simulink model "IPC"  (R2019b)
settings: Solver=FixedStepAuto  StartTime=0.0  StopTime=10  FixedStep=0.1  RelTol=1e-3
settings Model: Creator=JDALUZ1  LastModifiedBy=EMORAI12
settings SolverCC: PositivePriorityOrder=on  AutoInsertRateTranBlk=on  InsertRTBMode=Always
settings DebuggingCC: ArithmeticOperatorsInVariantConditions=warning
settings SFSimCC: CustomCodeUndefinedFunction=UseInterfaceOnly
settings CodeAppCC: StateflowObjectComments=on

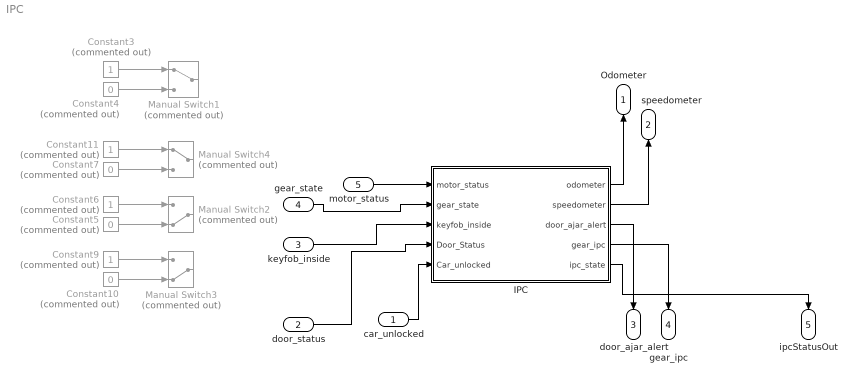
== system IPC ==
  car_unlocked : Inport
  door_status : Inport  Port=2
  keyfob_inside : Inport  Port=3
  gear_state : Inport  Port=4
  motor_status : Inport  Port=5
  Constant{4..5,7,10} (4 alike) : Constant  Commented=on  Value=0
  Constant{3,6,9,11} (4 alike) : Constant  Commented=on
  IPC : Stateflow chart  TreatAsAtomicUnit=on
  Manual Switch1 : ManualSwitch  Commented=on
  Manual Switch2 : ManualSwitch  Commented=on  CurrentSetting=0
  Manual Switch3 : ManualSwitch  Commented=on  CurrentSetting=0
  Manual Switch4 : ManualSwitch  Commented=on
  Odometer : Outport
  speedometer : Outport  Port=2
  door_ajar_alert : Outport  Port=3
  gear_ipc : Outport  Port=4
  ipcStatusOut : Outport  Port=5
  wires:
  IPC/2(speedometer) -> speedometer/1
  IPC/1(odometer) -> Odometer/1
  IPC/3(door_ajar_alert) -> door_ajar_alert/1
  Constant3/1 -> Manual Switch1/1
  Constant4/1 -> Manual Switch1/2
  gear_state/1 -> IPC/2(gear_state)
  IPC/4(gear_ipc) -> gear_ipc/1
  Constant9/1 -> Manual Switch3/1
  Constant10/1 -> Manual Switch3/2
  Constant5/1 -> Manual Switch2/2
  Constant6/1 -> Manual Switch2/1
  Constant7/1 -> Manual Switch4/2
  Constant11/1 -> Manual Switch4/1
  car_unlocked/1 -> IPC/5(Car_unlocked)
  door_status/1 -> IPC/4(Door_Status)
  keyfob_inside/1 -> IPC/3(keyfob_inside)
  motor_status/1 -> IPC/1(motor_status)
  IPC/5(ipc_state) -> ipcStatusOut/1

== stateflow chart IPC/IPC ==
  state door_lock_and_closed
    entry:
    gear_ipc=0;% marcha do carro em default
    door_ajar_alert=0 %led de alerta desligado
    lock_unlock=0; %porta trancada
    ipc_state=0;      %painel desligado
    speedometer=0;%speedomer na origem
    odometer=0; %odometer na origem
    %motor_status=0;%motor não está operando
    during:
    if(motor_status==0 )%se motor desligado
    if (Door_Status==1&&Car_unlocked==0) %se porta aberta e destravada
    ipc_state=1;  %liga o painel
    door_ajar_alert=1;  %liga led de alerta
    elseif (Door_Status==0) %se porta fechada
    door_ajar_alert=0; %n liga led de alerta
    end
    end
  note: % testa se o chaveiro foi acionado (destrava) e se a chave está fora do carro e se o motor está off
  state door_unlock_and_open
    entry:
    lock_unlock=1;
    during:
    if (Door_Status==1 )
    if (keyfob_inside==1)
    ipc_state=1;
    else
    ipc_state=0;
    end
    %gear_ipc=gear_state%status da marcha do carro
    door_ajar_alert=1;
    elseif (Door_Status==0)
    door_ajar_alert=0;
    if (keyfob_inside==1)
    ipc_state=1;
    else
    ipc_state=0;
    end
    end
  note: % testa se a chave está dentro do carro , se a partida do motor foi concluida com exito e se as portas foram fechadas.
  state SWEEP_ON
    en,du:
    if (cont==22)
    odometer=odometer+1;
    cont=1;
    end
    speedometer=speedometer+1;
    cont=cont+1;
    gear_ipc=gear_state%status da marcha do carro
    on after (500,msec):
    exit:
    cont=1;
  state wellcome_and_panel_indicators_on
    entry:
    ipc_state=1; %painel ligado
    %gear_ipc=gear_state%status da marcha do carro
    speedometer=0;%speedomer na origem
    odometer=0; %odometer na origem
    %motor_status=1;
    exit:
    cont=1;
  note: % testa se a chave está dentro do carro ,se a porta está fechada, se a partida do motor foi concluida com exito e se o motor ligou
  note: % testa se o chaveiro foi acionado (trancar) e se o motor continua desligado
  state SWEEP_OFF
    en,du:
    if (cont==22)
    odometer=odometer-1;
    cont=1;
    end
    speedometer=speedometer-1;
    cont=cont+1;
    gear_ipc=gear_state;%status da marcha do carro
    on after (500,msec):
  state IPC_DRIVING
    en,du:
    gear_ipc=gear_state%status da marcha do carro
    speedometer=0;
    odometer=2;
    if (Door_Status==1) %se porta aberta e destravada
    ipc_state=1;  %liga o painel
    door_ajar_alert=1;  %liga led de alerta
    elseif (Door_Status==0) %se porta fechada
    door_ajar_alert=0; %n liga led de alerta
    end
  note: % testa se se a parada do motor foi concluida com exito e se o motor foi desligado
  (default) -> door_lock_and_closed
  door_lock_and_closed -> door_unlock_and_open : [Car_unlocked==1 && motor_status==0 ]
  door_unlock_and_open -> wellcome_and_panel_indicators_on [order 2] : [ motor_status==1]
  door_unlock_and_open -> door_lock_and_closed [order 1] : [Car_unlocked==0 && motor_status==0 ]
  wellcome_and_panel_indicators_on -> SWEEP_ON
  SWEEP_ON -> SWEEP_OFF : [speedometer==220 && odometer==10]
  IPC_DRIVING -> door_lock_and_closed : [ motor_status==0 ]
  SWEEP_OFF -> IPC_DRIVING : [after(2,sec)&&speedometer==0 && odometer==0 ]
  data: odometer output; speedometer output; door_ajar_alert output; motor_status input; lock_unlock local; gear_ipc output; gear_state input; cont local; keyfob_inside input; Door_Status input; Car_unlocked input; ipc_state output
